simulink model "MilTesting"  (R2020b)
settings: Solver=VariableStepAuto  StartTime=0.0  StopTime=10.0  RelTol=1e-3
undefined symbols (not defined in the file or in its folder): sigbuilder_block
settings Model: Creator=99003785  LastModifiedBy=99003785

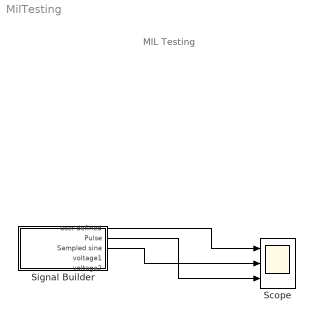
== system MilTesting ==
  note: MIL Testing
  Scope : Scope  NumInputPorts=3
  Signal Builder : Subsystem  Tag=STV Subsys  LoadFcn=sigbuilder_block('load');  StartFcn=sigbuilder_block('start');  StopFcn=sigbuilder_block('stop');  ClipboardFcn=sigbuilder_block('clipboard');  mask(Sigbuilder block){tuvar=[0:10]}
      mask help: Simulink:masks:SigbuilderBlock_MD
      mask init:
      | if ~strcmp(get_param(bdroot(gcbh),'SimulationStatus'),'stopped') tuvar = sigbuilder_block('maskInit'); end
      settings: CopyFcn=sigbuilder_block('copy');  DeleteFcn=sigbuilder_block('delete');  ModelCloseFcn=sigbuilder_block('modelClose');  PreSaveFcn=sigbuilder_block('preSave');  PauseFcn=sigbuilder_block('pause');  ContinueFcn=sigbuilder_block('continue');  NameChangeFcn=sigbuilder_block('namechange');  OpenFcn=sigbuilder_block('open',[777.75 115.5 550.5 399.75 ]);  CloseFcn=sigbuilder_block('close');
      mask Display: plot(0, 0, 100, 100,[2, 2, 32, 32, 2], [68, 8, 8, 68, 68],[32, 2], [38, 38], [32, 19, 2],[53, 60, 44], [32, 17, 17, 2],[16, 16, 31, 31]);txt = getActiveGroup(gcbh);text(2, 100, txt,'verticalAlignment', 'top');
  wires:
  Signal Builder/2(Pulse) -> Scope/3
  Signal Builder/1(user defined) -> Scope/1
  Signal Builder/3(Sampled sine) -> Scope/2

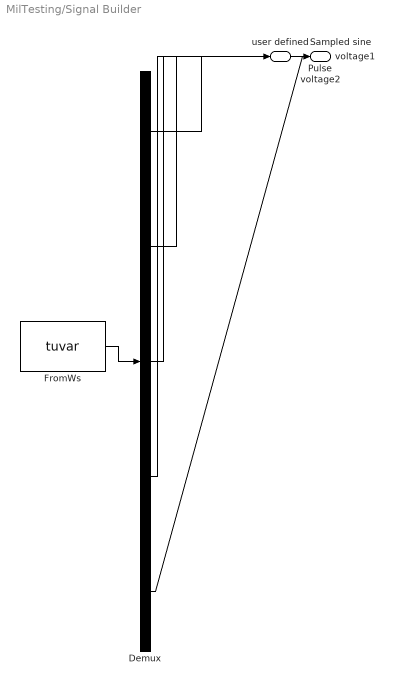
== system MilTesting/Signal Builder ==
  Demux : Demux  Tag=STV Demux  Outputs=5
      settings: DisplayOption=none
  FromWs : FromWorkspace  Tag=STV FromWs  VariableName=tuvar
      SigBuilderData=|
      | common.afterFinalStr = 'Extrapolate'
      | common.sampleTime = 0
      | dataSet.timeRange = [0 10]
      | dataSet.name = 'Group 1'
      | sbobj.Groups.Name = 'Group 1'
      | sbobj.Groups.Signals(1).Name = 'user defined'
      | sbobj.Groups.Signals(1).XData = [0 3.98 4 4 4.58 5.08 6 6 10]
      | sbobj.Groups.Signals(1).YData = [0 0 0 0.38 0.554537037037 0.41 0.615 0 0]
      | sbobj.Groups.Signals(2).Name = 'Pulse'
      | sbobj.Groups.Signals(2).XData = [0 4 4 6 6 10]
      | sbobj.Groups.Signals(2).YData = [0 0 1 1 0 0]
      | sbobj.Groups.Signals(3).Name = 'Sampled sine'
      | sbobj.Groups.Signals(3).XData = [0 0.125 0.25 0.375 0.5 0.625 0.75 0.875 1 1.125 1.25 1.375 1.5 1.625 1.75 1.875 2 2.125 2.25 2.375 2.5 2.625 2.75 2.875 3 3.125 3.25 3.375 3.5 3.625 3.75 3.875 4 4.125 4.25 4.375 4.5 4.625 4.75 4.875 5 5.125 5.25 5.375 5.5 5.625 5.75 5.875 6 6.125 6.25 6.375 6.5 6.625 6.75 6.875 7 7.125 7.25 7.375 7.5 7.625 7.75 7.875 8 8.125 8.25 8.375 8.5 8.625 8.75 8.875 9 9.125 9.25 9.375 9.5 9.625 9.75 9.875 10]
      | sbobj.Groups.Signals(3).YData = [1 2.41421356237 3 2.41421356237 1 -0.414213562373 -1 -0.414213562373 1 2.41421356237 3 2.41421356237 1 -0.414213562373 -1 -0.414213562373 1 2.1 3 2.41421356237 1 -0.414213562373 -1 -0.414213562373 1 2.41421356237 3 2.41421356237 1 -0.414213562373 -1 -0.414213562373 1 2.41421356237 3 2.41421356237 1 -0.414213562373 -1 -0.414213562373 1 2.41421356237 3 2.41421356237 1 -0.414213562373 -1 -0.414213562373 1 2.41421356237 3 2.41421356237 1 -0.414213562373 -1 -0.414213562373 1 2.41421356237 3 2.41421356237 1 -0.414213562373 -1 -0.414213562373 1 2.41421356237 3 2.41421356237 1 -0.414213562373 -1 -0.414213562373 1 2.41421356237 3 2.41421356237 1 -0.414213562373 -1 -0.414213562373 1]
      | sbobj.Groups.Signals(4).Name = 'voltage1'
      | sbobj.Groups.Signals(4).XData = [0 1 2 3 4 5 6 7 8 9 10 11 12 13]
      | sbobj.Groups.Signals(4).YData = [10 20 21 43 24 26 35 27 34 33 19 21 30 34]
      | sbobj.Groups.Signals(5).Name = 'voltage2'
      | sbobj.Groups.Signals(5).XData = [0 1 2 3 4 5 6 7 8 9 10 11 12 13]
      | sbobj.Groups.Signals(5).YData = [43 21 20 20 19 17 32 26 20 24 24 25 11 12]
  user defined : Outport  Tag=STV Outport
  Pulse : Outport  Tag=STV Outport  Port=2
  Sampled sine : Outport  Tag=STV Outport  Port=3
  voltage1 : Outport  Tag=STV Outport  Port=4
  voltage2 : Outport  Tag=STV Outport  Port=5
  wires:
  Demux/1 -> user defined/1
  FromWs/1 -> Demux/1
  Demux/2 -> Pulse/1
  Demux/3 -> Sampled sine/1
  Demux/4 -> voltage1/1
  Demux/5 -> voltage2/1
